simulink model "Domek_"  (R2018a)
settings: Solver=VariableStepAuto  StartTime=0.0  StopTime=1000  RelTol=1e-3
values from neighbouring files (symbols this model uses):
  cp = 1000    [domek.m]
  cv_p = 24000    [domek.m]
  cv_w = 48000    [domek.m]
  fpN = 0.1    [domek.m]
  fpn = fpN    (= 0.1)    [domek.m]
  K1 = C(1,1)    [domek.m]
  Kp = p*Kw    [domek.m]
  Kw = C(2,1)    [domek.m]
  ro_p = 1.2    [domek.m]
  Tz = TzN + dTz    (= 75)    [domek.m]
  Tzew = TzewN +dT    (= -17)    [domek.m]
  TzewN = -22    [domek.m]
  TzN = 80    [domek.m]
  War_Tp = T(2,1)    [domek.m]
  War_Twew = T(1,1)    [domek.m]
settings Model: Creator=stasz  LastModifiedBy=stasz
settings DebuggingCC: LibraryContextMissingDiagnostic=warning
settings SFSimCC: SimUseLocalCustomCode=on
settings RTWCC: RTWUseLocalCustomCode=on

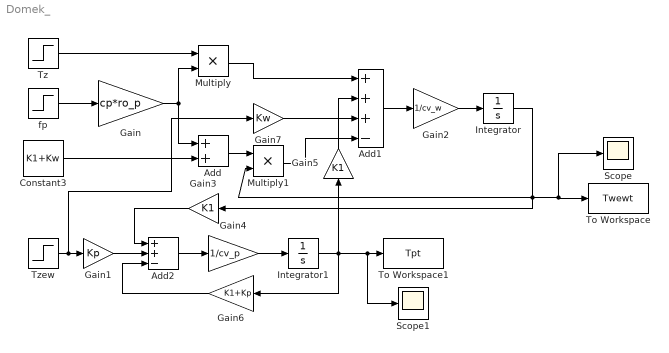
== system Domek_ ==
  Add : Sum
  Add1 : Sum  Inputs=+++-
  Add2 : Sum  Inputs=++-
  Constant3 : Constant  Value=K1+Kw
  Gain : Gain  Gain=cp*ro_p
  Gain1 : Gain  Gain=Kp
  Gain2 : Gain  Gain=1/cv_w
  Gain3 : Gain  Gain=K1
  Gain4 : Gain  Gain=1/cv_p
  Gain5 : Gain  Gain=K1
  Gain6 : Gain  Gain=K1+Kp
  Gain7 : Gain  Gain=Kw
  Integrator : Integrator  InitialCondition=War_Twew
  Integrator1 : Integrator  InitialCondition=War_Tp
  Multiply : Product
  Multiply1 : Product
  Scope : Scope
  Scope1 : Scope
  To Workspace : ToWorkspace  VariableName=Twewt  SaveFormat=Timeseries  SampleTime=-1
  To Workspace1 : ToWorkspace  VariableName=Tpt  SaveFormat=Timeseries  SampleTime=-1
  "Tz " : Step  Before=TzN  After=Tz  SampleTime=0
  Tzew : Step  Before=TzewN  After=Tzew  SampleTime=0
  fp : Step  Before=fpN  After=fpn  SampleTime=0
  wires:
  Integrator1/1 -> Gain6/1, Scope1/1, To Workspace1/1, Gain5/1
  Gain6/1 -> Add2/3
  Gain3/1 -> Add2/1
  Constant3/1 -> Add/2
  Add2/1 -> Gain4/1
  Multiply/1 -> Add1/1
  Multiply1/1 -> Add1/4
  Gain5/1 -> Add1/2
  Gain1/1 -> Add2/2
  Integrator/1 -> Gain3/1, Scope/1, To Workspace/1, Multiply1/2
  Tzew/1 -> Gain7/1, Gain1/1
  Add/1 -> Multiply1/1
  "Tz "/1 -> Multiply/1
  Add1/1 -> Gain2/1
  Gain2/1 -> Integrator/1
  Gain/1 -> Add/1, Multiply/2
  Gain4/1 -> Integrator1/1
  fp/1 -> Gain/1
  Gain7/1 -> Add1/3
